simulink model "QRotorSimulation"  (R2023a)
settings: Solver=VariableStepAuto  StartTime=0.0  StopTime=100  RelTol=1e-9
values from neighbouring files (symbols this model uses):
  A = [-skew(Oc),   eye(3),        -skew(Vc), zeros(3), zeros(3,4) ... (first row only)    [diff_q.m]    (also in model_LQR_Obsever.m)
  B = [   [0;0;0],zeros(3) ... (first row only)    [diff_q.m]    (also in model_LQR_Obsever.m)
  C = [    eye(3),   zeros(3), zeros(3),  zeros(3),zeros(3,4) ... (first row only)    [diff_q.m]    (also in model_LQR_Obsever.m)
  k = lqr(A, B, Q, R)    [model_LQR_Obsever.m]
  k1 = lqr(A1, B1, Q1, R)    [diff_q.m]    (also in model_LQR_Obsever.m)
  L_acker = (place(A',C', desired_poles))'    [diff_q.m]    (also in model_LQR_Obsever.m)
  target_pos = [1,1,1]    [diff_q.m]
libraries: robotcorelib x1, uavutilslib x1
settings Model: PacingRate=79  Creator=carlossilvestre  LastModifiedBy=ADMIN
settings SolverCC: AlgebraicLoopSolver=TrustRegion
settings OptimizationCC: ReuseModelBlockBuffer=off
settings DebuggingCC: UnconnectedInputMsg=warning  UnconnectedOutputMsg=warning  UnconnectedLineMsg=warning
settings ModelReferenceCC: EnableRefExpFcnMdlSchedulingChecks=on

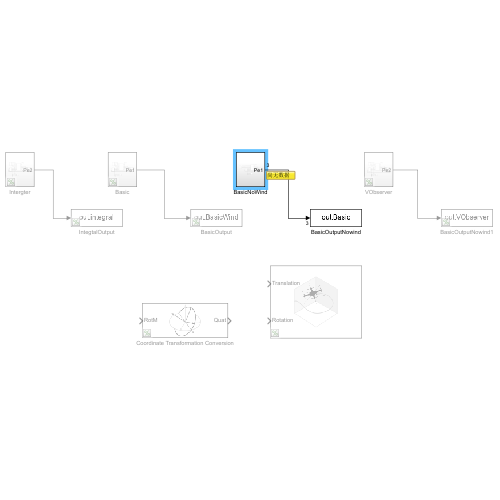
[thumbnail: Simulink's stored preview of the top-level diagram]
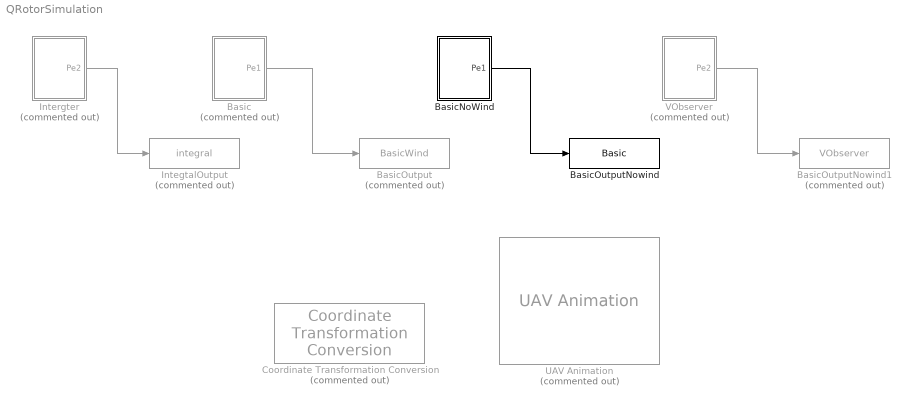
== system QRotorSimulation ==
  Basic : Subsystem  Commented=on
  BasicNoWind : Subsystem
  BasicOutput : ToWorkspace  Commented=on  VariableName=BasicWind  SaveFormat=Timeseries  SampleTime=-1
  BasicOutputNowind : ToWorkspace  VariableName=Basic  SaveFormat=Timeseries  SampleTime=-1
  BasicOutputNowind1 : ToWorkspace  Commented=on  VariableName=VObserver  SaveFormat=Timeseries  SampleTime=-1
  Coordinate Transformation Conversion : robotcorelib/Coordinate Transformation Conversion  Commented=on  InputRepresentation=Rotation Matrix  InputEulerSequence=ZYX  ShowTrVecInputPort=on  OutputRepresentation=Quaternion  OutputEulerSequence=ZYX  ShowTrVecOutputPort=on  SimulateUsing=Interpreted execution
      settings: LibrarySourceBlock=uavutilslib/Coordinate Transformation Conversion
  IntegtalOutput : ToWorkspace  Commented=on  VariableName=integral  SaveFormat=Timeseries  SampleTime=-1
  Intergter : Subsystem  Commented=on
  UAV Animation : uavutilslib/UAV Animation  Commented=on  UAVType=Multirotor  UAVSize=1  InertialZDirection=Down  SampleTime=-1
  VObserver : Subsystem  Commented=on
  wires:
  Intergter/1(Pe2) -> IntegtalOutput/1
  Basic/1(Pe1) -> BasicOutput/1
  BasicNoWind/1(Pe1) -> BasicOutputNowind/1
  VObserver/1(Pe2) -> BasicOutputNowind1/1

== system QRotorSimulation/Basic ==
  Constant : Constant  Value=k1
  Controller : Subsystem
  Demux : Demux  Outputs=3
  Nonlinear Transformation : MATLAB Function  TreatAsAtomicUnit=on
  Quardrotor : Subsystem
  Target Generator : Subsystem
  Ve : Scope
  XY Graph : Record  FileSettingsInternal="{\"entries\":[{\"content\":{\"excelSettings\":{\"content\":{},\"type\":\"Streamout.ExcelSettings\"}},\"type\":\"Streamout.FileSettingStorage\",\"uuid\":\"0487771f-67df-4d95-832c-7bf71d09cbca\"}],\"packageUris\":[\"http://schema.mathworks.com/mf0/streamout_blocks/R2020a\"],\"version\":\"1.0\"}"  Layout=[1 1]  SignalsInternal="{\"entries\":[{\"content\":{\"signals\":[{\"content\":{\"blockPath\":[\"QRotorSimulation/Basic/XY Graph\"],\"dimensions\":[1],\"domain\":\"QRotorSimulation/Basic/XY Graph\",\"lineColor\":\"#d95319\",\"port\":1,\"signalID\":1086,\"signalName\":\"Demux:1\"},\"type\":\"RecordBlkView.Signal\",\"uuid\":\"f90e91e6-e4ac-4811-9662-c694516e1994\"},{\"content\":{\"blockPath\":[\"QRotorSimulation/Basic/XY Graph\"],\"dimensions\":[1],\"domain\":\"QRotorSimulation/Basic/XY Graph\",\"lineColor\":\"#edb120\",\"port\":2,\"signalID\":1089,\"signalName\":\"Demux:2\"},\"type\":\"RecordBlkView.Signal\",\"uuid\":\"4a6e3aa6-85d4-4a9f-a4ee-96b742c40e35\"}]},\"type\":\"RecordBlkView.InputSignals\",\"uuid\":\"6a15db31-b281-48b1-89f1-5f9fae2ff927\"}],\"packageUris\":[\"http://schema.mathworks.com/mf0/streamout_blocks/R2020a\"],\"version\":\"1.0\"}"  VisualizationBindings="{\"xyplotplugin\":{\"info\":[{\"series\":[],\"subplotID\":1}]}}"  CompatibilityTag=XY
  Pe1 : Outport
  wires:
  Quardrotor/1(P) -> Demux/1, Pe1/1, Nonlinear Transformation/5(P)
  Quardrotor/3(Omega) -> Nonlinear Transformation/7(Omega)
  Nonlinear Transformation/3(Le) -> Controller/3(Le)
  Constant/1 -> Controller/5(k)
  Controller/2(T) -> Quardrotor/2(Thrust)
  Target Generator/4(Omega C) -> Nonlinear Transformation/3(OmeagC)
  Target Generator/5(R C) -> Nonlinear Transformation/4(Rc)
  Nonlinear Transformation/4(Pe) -> Controller/4(Pe)
  Nonlinear Transformation/1(Ve) -> Ve/1, Controller/1(Ve)
  Target Generator/2(Velocity C) -> Nonlinear Transformation/2(Vc)
  Quardrotor/2(V) -> Nonlinear Transformation/6(V)
  Nonlinear Transformation/2(Oe) -> Controller/2(Oe)
  Controller/1(n) -> Quardrotor/1(Torque)
  Target Generator/1(Position C) -> Nonlinear Transformation/1(Pc)
  Demux/2 -> XY Graph/2
  Demux/1 -> XY Graph/1
  Quardrotor/4(R) -> Nonlinear Transformation/8(R)

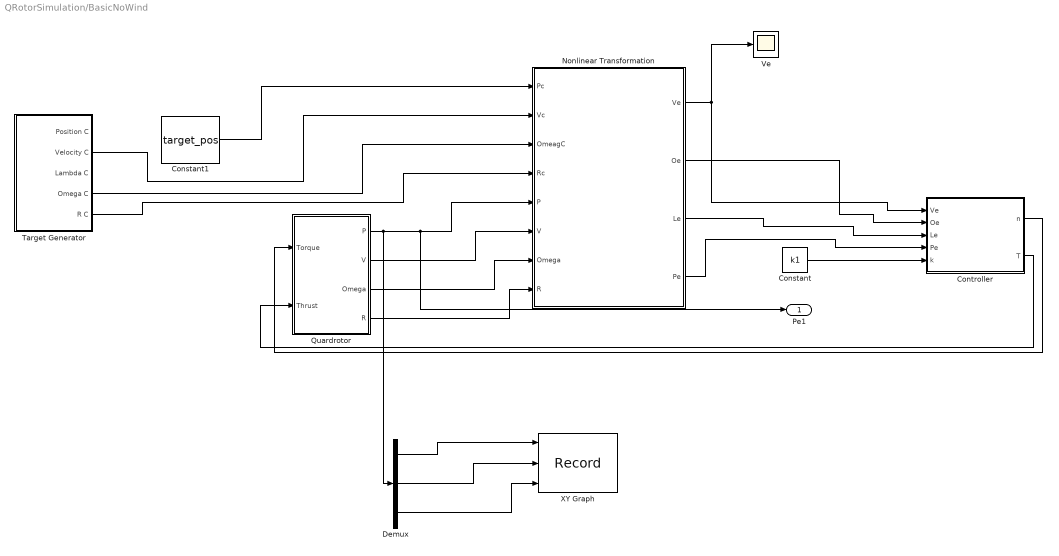
== system QRotorSimulation/BasicNoWind ==
  Constant : Constant  Value=k1
  Constant1 : Constant  Value=target_pos
  Controller : Subsystem
  Demux : Demux  Outputs=3
  Nonlinear Transformation : MATLAB Function  TreatAsAtomicUnit=on
  Quardrotor : Subsystem
  Target Generator : Subsystem
  Ve : Scope
  XY Graph : Record  FileSettingsInternal="{\"entries\":[{\"content\":{\"excelSettings\":{\"content\":{},\"type\":\"Streamout.ExcelSettings\"}},\"type\":\"Streamout.FileSettingStorage\",\"uuid\":\"6b954509-a0f9-4bc4-929f-937e6fe2c196\"}],\"packageUris\":[\"http://schema.mathworks.com/mf0/streamout_blocks/R2020a\"],\"version\":\"1.0\"}"  Layout=[1 1]  SignalsInternal="{\"entries\":[{\"content\":{\"signals\":[{\"content\":{\"blockPath\":[\"QRotorSimulation/BasicNoWind/XY Graph\"],\"dimensions\":[1],\"domain\":\"QRotorSimulation/BasicNoWind/XY Graph\",\"lineColor\":\"#77ac30\",\"port\":1,\"sid\":[\"\"],\"signalID\":3826,\"signalName\":\"Demux:1\"},\"type\":\"RecordBlkView.Signal\",\"uuid\":\"1b7d485a-109d-4aad-9f55-56817bc70bf2\"},{\"content\":{\"blockPath\":[\"QRotorSimulation/BasicNoWind/XY Graph\"],\"dimensions\":[1],\"domain\":\"QRotorSimulation/BasicNoWind/XY Graph\",\"lineColor\":\"#4dbeee\",\"port\":2,\"sid\":[\"\"],\"signalID\":3830,\"signalName\":\"Demux:2\"},\"type\":\"RecordBlkView.Signal\",\"uuid\":\"83925266-2204-43e3-9e67-c8fa90e0486b\"},{\"content\":{\"blockPath\":[\"QRotorSimulation/BasicNoWind/XY Graph\"],\"dimensions\":[1],\"domain\":\"QRotorSimulation/BasicNoWind/XY Graph\",\"lineColor\":\"#a2142f\",\"port\":3,\"sid\":[\"\"],\"signalID\":3834,\"signalName\":\"Demux:3\"},\"type\":\"RecordBlkView.Signal\",\"uuid\":\"81f905cc-e198-402a-a94e-d97bcbf9668d\"}]},\"type\":\"RecordBlkView.InputSignals\",\"uuid\":\"1cf66a60-863d-452f-b7c5-5f047e404abc\"}],\"packageUris\":[\"http://schema.mathworks.com/mf0/streamout_blocks/R2020a\"],\"version\":\"1.0\"}"  VisualizationBindings="{\"xyplotplugin\":{\"info\":[{\"series\":[],\"subplotID\":1}]}}"  CompatibilityTag=XY
  Pe1 : Outport
  wires:
  Quardrotor/4(R) -> Nonlinear Transformation/8(R)
  Demux/1 -> XY Graph/1
  Demux/2 -> XY Graph/2
  Controller/1(n) -> Quardrotor/1(Torque)
  Nonlinear Transformation/2(Oe) -> Controller/2(Oe)
  Quardrotor/2(V) -> Nonlinear Transformation/6(V)
  Target Generator/2(Velocity C) -> Nonlinear Transformation/2(Vc)
  Nonlinear Transformation/1(Ve) -> Controller/1(Ve), Ve/1
  Nonlinear Transformation/4(Pe) -> Controller/4(Pe)
  Target Generator/5(R C) -> Nonlinear Transformation/4(Rc)
  Target Generator/4(Omega C) -> Nonlinear Transformation/3(OmeagC)
  Controller/2(T) -> Quardrotor/2(Thrust)
  Constant/1 -> Controller/5(k)
  Nonlinear Transformation/3(Le) -> Controller/3(Le)
  Quardrotor/3(Omega) -> Nonlinear Transformation/7(Omega)
  Quardrotor/1(P) -> Pe1/1, Nonlinear Transformation/5(P), Demux/1
  Demux/3 -> XY Graph/3
  Constant1/1 -> Nonlinear Transformation/1(Pc)

== system QRotorSimulation/Intergter ==
  Constant : Constant  Value=k
  Controller : Subsystem
  Demux : Demux  Outputs=3
  Nonlinear Transformation : MATLAB Function  TreatAsAtomicUnit=on
  Pe : Scope
  Quardrotor : Subsystem
  Target Generator : Subsystem
  Ve : Scope
  XY Graph : Record  FileSettingsInternal="{\"entries\":[{\"content\":{\"excelSettings\":{\"content\":{},\"type\":\"Streamout.ExcelSettings\"}},\"type\":\"Streamout.FileSettingStorage\",\"uuid\":\"5274d8c0-192d-4b89-88ac-329a06cc1ef7\"}],\"packageUris\":[\"http://schema.mathworks.com/mf0/streamout_blocks/R2020a\"],\"version\":\"1.0\"}"  Layout=[1 1]  SignalsInternal="{\"entries\":[{\"content\":{\"signals\":[{\"content\":{\"blockPath\":[\"QRotorSimulation/Intergter/XY Graph\"],\"dimensions\":[1],\"domain\":\"QRotorSimulation/Intergter/XY Graph\",\"lineColor\":\"#64d413\",\"port\":1,\"signalID\":1070,\"signalName\":\"Demux:1\"},\"type\":\"RecordBlkView.Signal\",\"uuid\":\"1ff87784-21ca-461c-803a-48280af1891b\"},{\"content\":{\"blockPath\":[\"QRotorSimulation/Intergter/XY Graph\"],\"dimensions\":[1],\"domain\":\"QRotorSimulation/Intergter/XY Graph\",\"lineColor\":\"#ff13a6\",\"port\":2,\"signalID\":1073,\"signalName\":\"Demux:2\"},\"type\":\"RecordBlkView.Signal\",\"uuid\":\"24908c8c-4281-4163-98ae-854703be901d\"}]},\"type\":\"RecordBlkView.InputSignals\",\"uuid\":\"2df63969-910d-47c6-a209-6b5a32245b9d\"}],\"packageUris\":[\"http://schema.mathworks.com/mf0/streamout_blocks/R2020a\"],\"version\":\"1.0\"}"  VisualizationBindings="{\"xyplotplugin\":{\"info\":[{\"series\":[],\"subplotID\":1}]}}"  CompatibilityTag=XY
  Pe2 : Outport
  wires:
  Quardrotor/4(R) -> Nonlinear Transformation/8(R)
  Demux/1 -> XY Graph/1
  Demux/2 -> XY Graph/2
  Target Generator/1(Position C) -> Nonlinear Transformation/1(Pc)
  Controller/1(n) -> Quardrotor/1(Torque)
  Nonlinear Transformation/2(Oe) -> Controller/2(Oe)
  Quardrotor/2(V) -> Nonlinear Transformation/6(V)
  Target Generator/2(Velocity C) -> Nonlinear Transformation/2(Vc)
  Nonlinear Transformation/1(Ve) -> Controller/1(Ve), Ve/1
  Target Generator/5(R C) -> Nonlinear Transformation/4(Rc)
  Target Generator/4(Omega C) -> Nonlinear Transformation/3(OmeagC)
  Controller/2(T) -> Quardrotor/2(Thrust)
  Constant/1 -> Controller/5(k)
  Nonlinear Transformation/3(Le) -> Controller/3(Le)
  Quardrotor/3(Omega) -> Nonlinear Transformation/7(Omega)
  Quardrotor/1(P) -> Nonlinear Transformation/5(P), Pe2/1, Demux/1
  Nonlinear Transformation/4(Pe) -> Controller/4(Pe), Pe/1

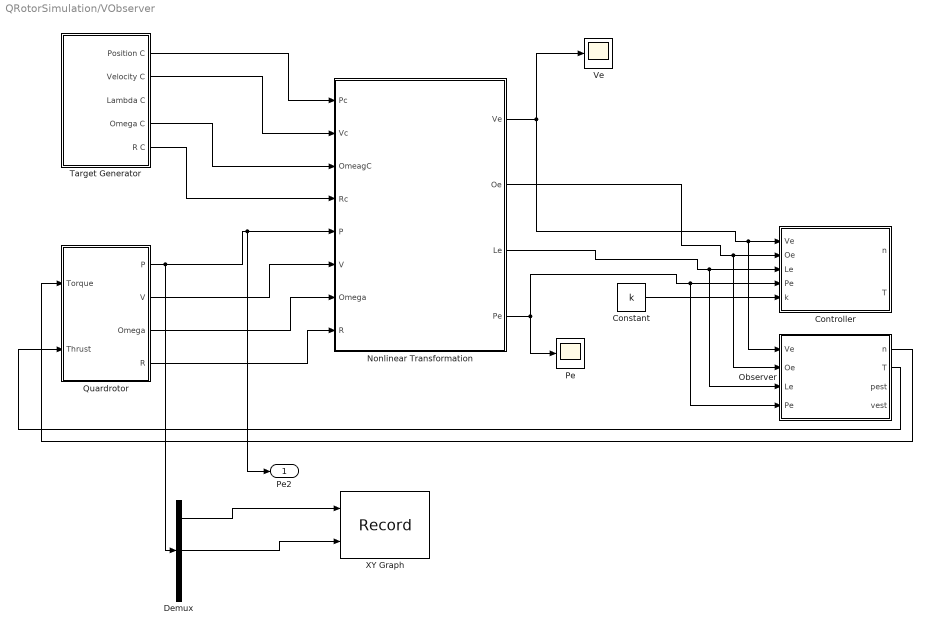
== system QRotorSimulation/VObserver ==
  Constant : Constant  Value=k
  Controller : Subsystem
  Demux : Demux  Outputs=3
  Nonlinear Transformation : MATLAB Function  TreatAsAtomicUnit=on
  Observer : Subsystem
  Pe : Scope
  Quardrotor : Subsystem
  Target Generator : Subsystem
  Ve : Scope
  XY Graph : Record  FileSettingsInternal="{\"entries\":[{\"content\":{\"excelSettings\":{\"content\":{},\"type\":\"Streamout.ExcelSettings\"}},\"type\":\"Streamout.FileSettingStorage\",\"uuid\":\"09f89506-ea5c-4e7c-be6e-909bc9330a96\"}],\"packageUris\":[\"http://schema.mathworks.com/mf0/streamout_blocks/R2020a\"],\"version\":\"1.0\"}"  Layout=[1 1]  SignalsInternal="{\"entries\":[{\"content\":{\"signals\":[{\"content\":{\"blockPath\":[\"QRotorSimulation/VObserver/XY Graph\"],\"dimensions\":[1],\"domain\":\"QRotorSimulation/VObserver/XY Graph\",\"lineColor\":\"#7e2f8e\",\"port\":1,\"signalID\":1062,\"signalName\":\"Demux:1\"},\"type\":\"RecordBlkView.Signal\",\"uuid\":\"913ab4c1-d204-4348-ad14-4cd9366a4f4d\"},{\"content\":{\"blockPath\":[\"QRotorSimulation/VObserver/XY Graph\"],\"dimensions\":[1],\"domain\":\"QRotorSimulation/VObserver/XY Graph\",\"lineColor\":\"#77ac30\",\"port\":2,\"signalID\":1065,\"signalName\":\"Demux:2\"},\"type\":\"RecordBlkView.Signal\",\"uuid\":\"1419c895-5134-46cb-881d-871a74845bf3\"}]},\"type\":\"RecordBlkView.InputSignals\",\"uuid\":\"c0c07795-0499-4d5b-ba90-fdcac508c0e4\"}],\"packageUris\":[\"http://schema.mathworks.com/mf0/streamout_blocks/R2020a\"],\"version\":\"1.0\"}"  VisualizationBindings="{\"xyplotplugin\":{\"info\":[{\"series\":[],\"subplotID\":1}]}}"  CompatibilityTag=XY
  Pe2 : Outport
  wires:
  Nonlinear Transformation/4(Pe) -> Pe/1, Observer/4(Pe), Controller/4(Pe)
  Quardrotor/1(P) -> Demux/1, Pe2/1, Nonlinear Transformation/5(P)
  Quardrotor/3(Omega) -> Nonlinear Transformation/7(Omega)
  Nonlinear Transformation/3(Le) -> Observer/3(Le), Controller/3(Le)
  Constant/1 -> Controller/5(k)
  Target Generator/4(Omega C) -> Nonlinear Transformation/3(OmeagC)
  Target Generator/5(R C) -> Nonlinear Transformation/4(Rc)
  Nonlinear Transformation/1(Ve) -> Ve/1, Observer/1(Ve), Controller/1(Ve)
  Target Generator/2(Velocity C) -> Nonlinear Transformation/2(Vc)
  Quardrotor/2(V) -> Nonlinear Transformation/6(V)
  Nonlinear Transformation/2(Oe) -> Observer/2(Oe), Controller/2(Oe)
  Target Generator/1(Position C) -> Nonlinear Transformation/1(Pc)
  Demux/2 -> XY Graph/2
  Demux/1 -> XY Graph/1
  Quardrotor/4(R) -> Nonlinear Transformation/8(R)
  Observer/1(n) -> Quardrotor/1(Torque)
  Observer/2(T) -> Quardrotor/2(Thrust)

== system QRotorSimulation/Basic/Controller ==
  Ve : Inport
  Oe : Inport  Port=2
  Le : Inport  Port=3
  Pe : Inport  Port=4
  k : Inport  Port=5
  Controller : MATLAB Function  TreatAsAtomicUnit=on
  n : Outport
  T : Outport  Port=2
  wires:
  Oe/1 -> Controller/2(Oe)
  Pe/1 -> Controller/4(Pe)
  Le/1 -> Controller/3(Le)
  Ve/1 -> Controller/1(Ve)
  Controller/2(n) -> n/1
  k/1 -> Controller/5(k)
  Controller/1(T) -> T/1

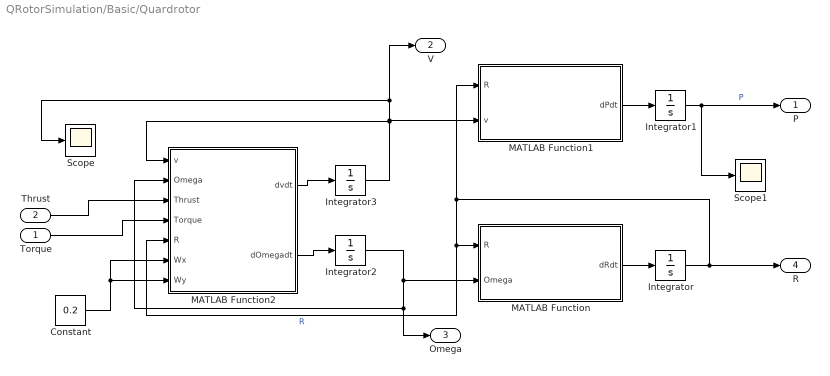
== system QRotorSimulation/Basic/Quardrotor ==
  Torque : Inport
  Thrust : Inport  Port=2  PortDimensions=1
  Constant : Constant  Value=0.2  VectorParams1D=off
  Integrator : Integrator  InitialCondition=eye(3)
  Integrator1 : Integrator  InitialCondition=[0,0,0]
  Integrator2 : Integrator  InitialCondition=[0,0,0]  ContinuousStateAttributes='omega'
  Integrator3 : Integrator  InitialCondition=[0,0,0]  ContinuousStateAttributes='velocity'
  MATLAB Function : MATLAB Function  TreatAsAtomicUnit=on
  MATLAB Function1 : MATLAB Function  TreatAsAtomicUnit=on
  MATLAB Function2 : MATLAB Function  TreatAsAtomicUnit=on
  Scope : Scope
  Scope1 : Scope
  P : Outport
  V : Outport  Port=2
  Omega : Outport  Port=3
  R : Outport  Port=4
  wires:
  Constant/1 -> MATLAB Function2/6(Wx), MATLAB Function2/7(Wy)
  Torque/1 -> MATLAB Function2/4(Torque)
  Thrust/1 -> MATLAB Function2/3(Thrust)
  Integrator/1 -> MATLAB Function/1(R), MATLAB Function2/5(R), MATLAB Function1/1(R), R/1  "R"
  MATLAB Function1/1(dPdt) -> Integrator1/1
  Integrator3/1 -> MATLAB Function2/1(v), MATLAB Function1/2(v), V/1, Scope/1
  MATLAB Function2/2(dOmegadt) -> Integrator2/1
  MATLAB Function/1(dRdt) -> Integrator/1
  Integrator2/1 -> MATLAB Function/2(Omega), MATLAB Function2/2(Omega), Omega/1
  Integrator1/1 -> P/1, Scope1/1  "P"
  MATLAB Function2/1(dvdt) -> Integrator3/1

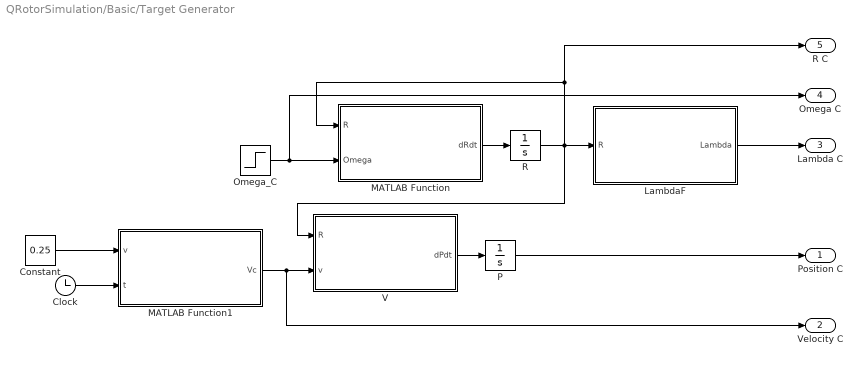
== system QRotorSimulation/Basic/Target Generator ==
  Clock : Clock
  Constant : Constant  Value=0.25
  LambdaF : MATLAB Function  TreatAsAtomicUnit=on
  MATLAB Function : MATLAB Function  TreatAsAtomicUnit=on
  MATLAB Function1 : MATLAB Function  TreatAsAtomicUnit=on
  Omega_C : Step  Time=0  Before=[0;0;0]  After=[0;0;0]  SampleTime=0
  P : Integrator
  R : Integrator  InitialCondition=eye(3)
  V : MATLAB Function  TreatAsAtomicUnit=on
  Position C : Outport
  Velocity C : Outport  Port=2
  Lambda C : Outport  Port=3
  Omega C : Outport  Port=4
  R C : Outport  Port=5
  wires:
  Clock/1 -> MATLAB Function1/2(t)
  Constant/1 -> MATLAB Function1/1(v)
  Omega_C/1 -> MATLAB Function/2(Omega), Omega C/1
  MATLAB Function1/1(Vc) -> V/2(v), Velocity C/1
  V/1(dPdt) -> P/1
  R/1 -> LambdaF/1(R), V/1(R), R C/1, MATLAB Function/1(R)
  MATLAB Function/1(dRdt) -> R/1
  P/1 -> Position C/1
  LambdaF/1(Lambda) -> Lambda C/1

== system QRotorSimulation/BasicNoWind/Controller ==
  Ve : Inport
  Oe : Inport  Port=2
  Le : Inport  Port=3
  Pe : Inport  Port=4
  k : Inport  Port=5
  Controller : MATLAB Function  TreatAsAtomicUnit=on
  n : Outport
  T : Outport  Port=2
  wires:
  Controller/1(T) -> T/1
  k/1 -> Controller/5(k)
  Controller/2(n) -> n/1
  Ve/1 -> Controller/1(Ve)
  Le/1 -> Controller/3(Le)
  Pe/1 -> Controller/4(Pe)
  Oe/1 -> Controller/2(Oe)

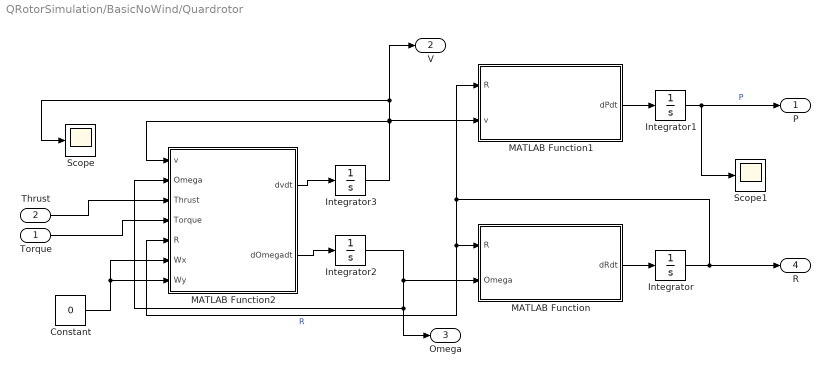
== system QRotorSimulation/BasicNoWind/Quardrotor ==
  Torque : Inport
  Thrust : Inport  Port=2  PortDimensions=1
  Constant : Constant  Value=0  VectorParams1D=off
  Integrator : Integrator  InitialCondition=eye(3)
  Integrator1 : Integrator  InitialCondition=[0,0,0]
  Integrator2 : Integrator  InitialCondition=[0,0,0]  ContinuousStateAttributes='omega'
  Integrator3 : Integrator  InitialCondition=[0,0,0]  ContinuousStateAttributes='velocity'
  MATLAB Function : MATLAB Function  TreatAsAtomicUnit=on
  MATLAB Function1 : MATLAB Function  TreatAsAtomicUnit=on
  MATLAB Function2 : MATLAB Function  TreatAsAtomicUnit=on
  Scope : Scope
  Scope1 : Scope
  P : Outport
  V : Outport  Port=2
  Omega : Outport  Port=3
  R : Outport  Port=4
  wires:
  MATLAB Function2/1(dvdt) -> Integrator3/1
  Integrator1/1 -> Scope1/1, P/1  "P"
  Integrator2/1 -> Omega/1, MATLAB Function2/2(Omega), MATLAB Function/2(Omega)
  MATLAB Function/1(dRdt) -> Integrator/1
  MATLAB Function2/2(dOmegadt) -> Integrator2/1
  Integrator3/1 -> Scope/1, V/1, MATLAB Function1/2(v), MATLAB Function2/1(v)
  MATLAB Function1/1(dPdt) -> Integrator1/1
  Integrator/1 -> R/1, MATLAB Function1/1(R), MATLAB Function2/5(R), MATLAB Function/1(R)  "R"
  Thrust/1 -> MATLAB Function2/3(Thrust)
  Torque/1 -> MATLAB Function2/4(Torque)
  Constant/1 -> MATLAB Function2/7(Wy), MATLAB Function2/6(Wx)

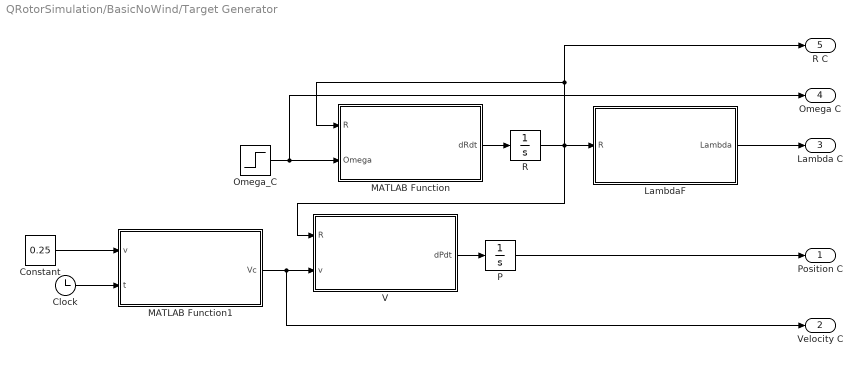
== system QRotorSimulation/BasicNoWind/Target Generator ==
  Clock : Clock
  Constant : Constant  Value=0.25
  LambdaF : MATLAB Function  TreatAsAtomicUnit=on
  MATLAB Function : MATLAB Function  TreatAsAtomicUnit=on
  MATLAB Function1 : MATLAB Function  TreatAsAtomicUnit=on
  Omega_C : Step  Time=0  Before=[0;0;0]  After=[0;0;0]  SampleTime=0
  P : Integrator
  R : Integrator  InitialCondition=eye(3)
  V : MATLAB Function  TreatAsAtomicUnit=on
  Position C : Outport
  Velocity C : Outport  Port=2
  Lambda C : Outport  Port=3
  Omega C : Outport  Port=4
  R C : Outport  Port=5
  wires:
  LambdaF/1(Lambda) -> Lambda C/1
  P/1 -> Position C/1
  MATLAB Function/1(dRdt) -> R/1
  R/1 -> MATLAB Function/1(R), R C/1, V/1(R), LambdaF/1(R)
  V/1(dPdt) -> P/1
  MATLAB Function1/1(Vc) -> Velocity C/1, V/2(v)
  Omega_C/1 -> Omega C/1, MATLAB Function/2(Omega)
  Constant/1 -> MATLAB Function1/1(v)
  Clock/1 -> MATLAB Function1/2(t)

== system QRotorSimulation/Intergter/Controller ==
  Ve : Inport
  Oe : Inport  Port=2
  Le : Inport  Port=3
  Pe : Inport  Port=4
  k : Inport  Port=5
  Controller : MATLAB Function  TreatAsAtomicUnit=on
  Int : MATLAB Function  TreatAsAtomicUnit=on
  Integrator : Integrator
  n : Outport
  T : Outport  Port=2
  wires:
  Controller/1(T) -> T/1
  k/1 -> Controller/6(k)
  Controller/2(n) -> n/1
  Integrator/1 -> Controller/5(Xi)
  Int/1(dXidt) -> Integrator/1
  Ve/1 -> Int/1(Ve), Controller/1(Ve)
  Le/1 -> Controller/3(Le), Int/3(Le)
  Pe/1 -> Controller/4(Pe), Int/4(Pe)
  Oe/1 -> Int/2(Oe), Controller/2(Oe)

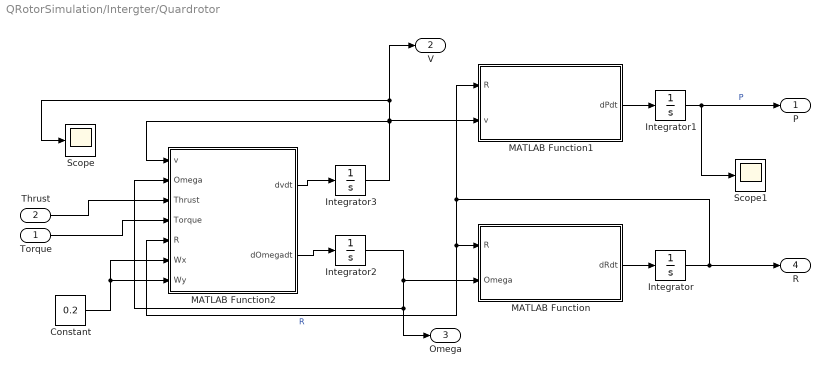
== system QRotorSimulation/Intergter/Quardrotor ==
  Torque : Inport
  Thrust : Inport  Port=2  PortDimensions=1
  Constant : Constant  Value=0.2
  Integrator : Integrator  InitialCondition=eye(3)
  Integrator1 : Integrator  InitialCondition=[0,0,0]
  Integrator2 : Integrator  InitialCondition=[0,0,0]  ContinuousStateAttributes='omega'
  Integrator3 : Integrator  InitialCondition=[0,0,0]  ContinuousStateAttributes='velocity'
  MATLAB Function : MATLAB Function  TreatAsAtomicUnit=on
  MATLAB Function1 : MATLAB Function  TreatAsAtomicUnit=on
  MATLAB Function2 : MATLAB Function  TreatAsAtomicUnit=on
  Scope : Scope
  Scope1 : Scope
  P : Outport
  V : Outport  Port=2
  Omega : Outport  Port=3
  R : Outport  Port=4
  wires:
  MATLAB Function2/1(dvdt) -> Integrator3/1
  Integrator1/1 -> Scope1/1, P/1  "P"
  Integrator2/1 -> Omega/1, MATLAB Function2/2(Omega), MATLAB Function/2(Omega)
  MATLAB Function/1(dRdt) -> Integrator/1
  MATLAB Function2/2(dOmegadt) -> Integrator2/1
  Integrator3/1 -> Scope/1, V/1, MATLAB Function1/2(v), MATLAB Function2/1(v)
  MATLAB Function1/1(dPdt) -> Integrator1/1
  Integrator/1 -> R/1, MATLAB Function1/1(R), MATLAB Function2/5(R), MATLAB Function/1(R)  "R"
  Thrust/1 -> MATLAB Function2/3(Thrust)
  Torque/1 -> MATLAB Function2/4(Torque)
  Constant/1 -> MATLAB Function2/7(Wy), MATLAB Function2/6(Wx)

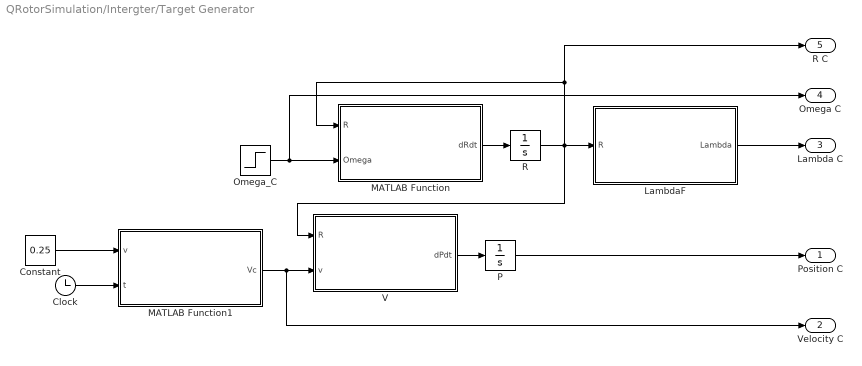
== system QRotorSimulation/Intergter/Target Generator ==
  Clock : Clock
  Constant : Constant  Value=0.25
  LambdaF : MATLAB Function  TreatAsAtomicUnit=on
  MATLAB Function : MATLAB Function  TreatAsAtomicUnit=on
  MATLAB Function1 : MATLAB Function  TreatAsAtomicUnit=on
  Omega_C : Step  Time=0  Before=[0;0;0]  After=[0;0;0]  SampleTime=0
  P : Integrator
  R : Integrator  InitialCondition=eye(3)
  V : MATLAB Function  TreatAsAtomicUnit=on
  Position C : Outport
  Velocity C : Outport  Port=2
  Lambda C : Outport  Port=3
  Omega C : Outport  Port=4
  R C : Outport  Port=5
  wires:
  LambdaF/1(Lambda) -> Lambda C/1
  P/1 -> Position C/1
  MATLAB Function/1(dRdt) -> R/1
  R/1 -> MATLAB Function/1(R), R C/1, V/1(R), LambdaF/1(R)
  V/1(dPdt) -> P/1
  MATLAB Function1/1(Vc) -> Velocity C/1, V/2(v)
  Omega_C/1 -> Omega C/1, MATLAB Function/2(Omega)
  Constant/1 -> MATLAB Function1/1(v)
  Clock/1 -> MATLAB Function1/2(t)

== system QRotorSimulation/VObserver/Controller ==
  Ve : Inport
  Oe : Inport  Port=2
  Le : Inport  Port=3
  Pe : Inport  Port=4
  k : Inport  Port=5
  Controller : MATLAB Function  TreatAsAtomicUnit=on
  Int : MATLAB Function  TreatAsAtomicUnit=on
  Integrator : Integrator
  n : Outport
  T : Outport  Port=2
  wires:
  Oe/1 -> Controller/2(Oe), Int/2(Oe)
  Pe/1 -> Int/4(Pe), Controller/4(Pe)
  Le/1 -> Int/3(Le), Controller/3(Le)
  Ve/1 -> Controller/1(Ve), Int/1(Ve)
  Int/1(dXidt) -> Integrator/1
  Integrator/1 -> Controller/5(Xi)
  Controller/2(n) -> n/1
  k/1 -> Controller/6(k)
  Controller/1(T) -> T/1

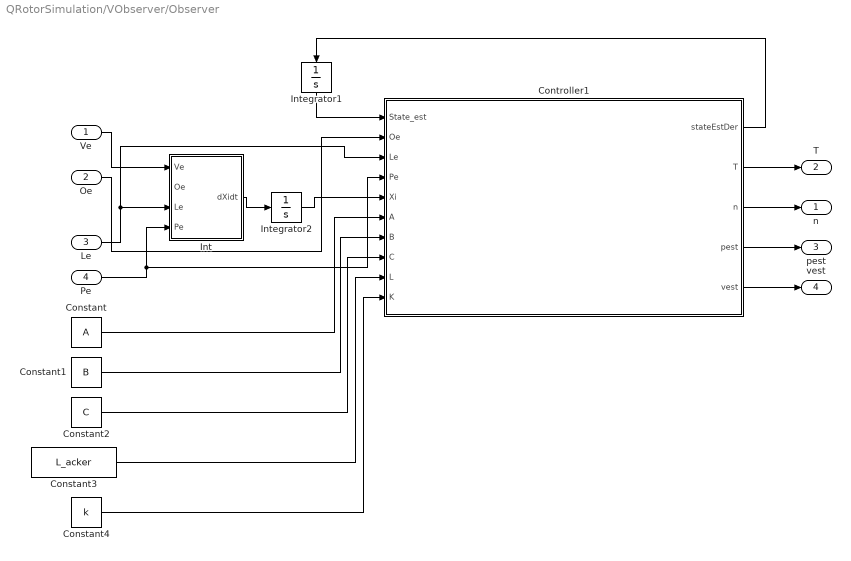
== system QRotorSimulation/VObserver/Observer ==
  Ve : Inport
  Oe : Inport  Port=2
  Le : Inport  Port=3
  Pe : Inport  Port=4
  Constant : Constant  Value=A
  Constant1 : Constant  Value=B
  Constant2 : Constant  Value=C
  Constant3 : Constant  Value=L_acker
  Constant4 : Constant  Value=k
  Controller1 : MATLAB Function  TreatAsAtomicUnit=on
  Int : MATLAB Function  TreatAsAtomicUnit=on
  Integrator1 : Integrator  InitialCondition=zeros(16,1)
  Integrator2 : Integrator
  n : Outport
  T : Outport  Port=2
  pest : Outport  Port=3
  vest : Outport  Port=4
  wires:
  Integrator1/1 -> Controller1/1(State_est)
  Controller1/1(stateEstDer) -> Integrator1/1
  Oe/1 -> Controller1/2(Oe)
  Pe/1 -> Controller1/4(Pe), Int/4(Pe)
  Le/1 -> Controller1/3(Le), Int/3(Le)
  Int/1(dXidt) -> Integrator2/1
  Controller1/2(T) -> T/1
  Controller1/3(n) -> n/1
  Constant/1 -> Controller1/6(A)
  Constant1/1 -> Controller1/7(B)
  Constant2/1 -> Controller1/8(C)
  Constant4/1 -> Controller1/10(K)
  Constant3/1 -> Controller1/9(L)
  Integrator2/1 -> Controller1/5(Xi)
  Controller1/5(vest) -> vest/1
  Controller1/4(pest) -> pest/1
  Ve/1 -> Int/1(Ve)

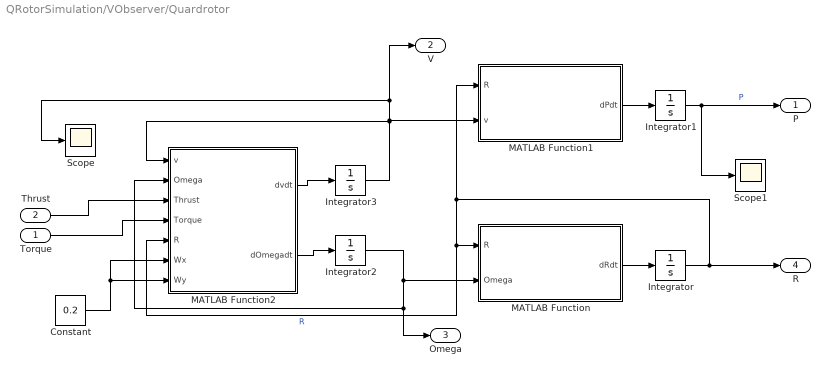
== system QRotorSimulation/VObserver/Quardrotor ==
  Torque : Inport
  Thrust : Inport  Port=2  PortDimensions=1
  Constant : Constant  Value=0.2
  Integrator : Integrator  InitialCondition=eye(3)
  Integrator1 : Integrator  InitialCondition=[0,0,0]
  Integrator2 : Integrator  InitialCondition=[0,0,0]  ContinuousStateAttributes='omega'
  Integrator3 : Integrator  InitialCondition=[0,0,0]  ContinuousStateAttributes='velocity'
  MATLAB Function : MATLAB Function  TreatAsAtomicUnit=on
  MATLAB Function1 : MATLAB Function  TreatAsAtomicUnit=on
  MATLAB Function2 : MATLAB Function  TreatAsAtomicUnit=on
  Scope : Scope
  Scope1 : Scope
  P : Outport
  V : Outport  Port=2
  Omega : Outport  Port=3
  R : Outport  Port=4
  wires:
  Constant/1 -> MATLAB Function2/6(Wx), MATLAB Function2/7(Wy)
  Torque/1 -> MATLAB Function2/4(Torque)
  Thrust/1 -> MATLAB Function2/3(Thrust)
  Integrator/1 -> MATLAB Function/1(R), MATLAB Function2/5(R), MATLAB Function1/1(R), R/1  "R"
  MATLAB Function1/1(dPdt) -> Integrator1/1
  Integrator3/1 -> MATLAB Function2/1(v), MATLAB Function1/2(v), V/1, Scope/1
  MATLAB Function2/2(dOmegadt) -> Integrator2/1
  MATLAB Function/1(dRdt) -> Integrator/1
  Integrator2/1 -> MATLAB Function/2(Omega), MATLAB Function2/2(Omega), Omega/1
  Integrator1/1 -> P/1, Scope1/1  "P"
  MATLAB Function2/1(dvdt) -> Integrator3/1

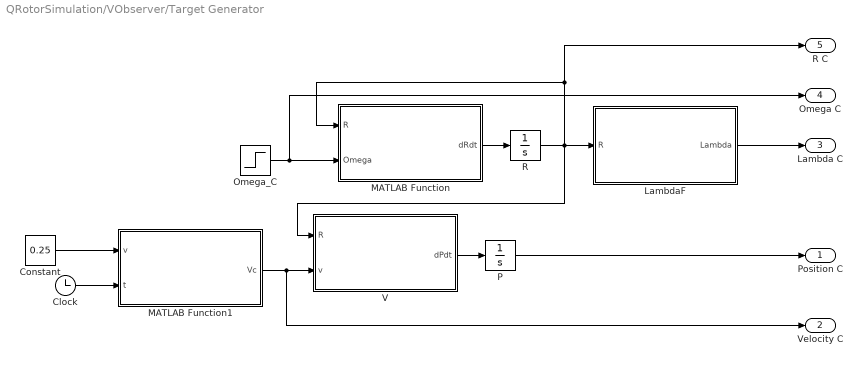
== system QRotorSimulation/VObserver/Target Generator ==
  Clock : Clock
  Constant : Constant  Value=0.25
  LambdaF : MATLAB Function  TreatAsAtomicUnit=on
  MATLAB Function : MATLAB Function  TreatAsAtomicUnit=on
  MATLAB Function1 : MATLAB Function  TreatAsAtomicUnit=on
  Omega_C : Step  Time=0  Before=[0;0;0]  After=[0;0;0]  SampleTime=0
  P : Integrator
  R : Integrator  InitialCondition=eye(3)
  V : MATLAB Function  TreatAsAtomicUnit=on
  Position C : Outport
  Velocity C : Outport  Port=2
  Lambda C : Outport  Port=3
  Omega C : Outport  Port=4
  R C : Outport  Port=5
  wires:
  Clock/1 -> MATLAB Function1/2(t)
  Constant/1 -> MATLAB Function1/1(v)
  Omega_C/1 -> MATLAB Function/2(Omega), Omega C/1
  MATLAB Function1/1(Vc) -> V/2(v), Velocity C/1
  V/1(dPdt) -> P/1
  R/1 -> LambdaF/1(R), V/1(R), R C/1, MATLAB Function/1(R)
  MATLAB Function/1(dRdt) -> R/1
  P/1 -> Position C/1
  LambdaF/1(Lambda) -> Lambda C/1

== matlab function QRotorSimulation/Intergter/Target Generator/MATLAB Function ==
  data: R input; dRdt output; Omega input
function dRdt = CompdRdt(R,Omega)
dRdt=R*skew(Omega);
end

== matlab function QRotorSimulation/Intergter/Target Generator/MATLAB Function1 ==
  data: v input; Vc output; t input
function Vc = VcGen(v,t)
Vc = [0;0;0];

if(t>10)
    Vc = [v;0;0];
end
if(t>30)
    Vc = [0;v;0];
end

if(t>50)
    Vc = [-v;0;0];
end

if(t>70)
    Vc = [0;-v;0]; 
end

if(t>90)
    Vc = [0;0;0]; %stop
end

end

== matlab function QRotorSimulation/Basic/Controller/Controller ==
  data: Ve input; Oe input; Le input; Pe input; T output; n output; k input
function [T,n] = Controller(Ve,Oe,Le,Pe,k)

State = [Pe; Ve; Le; Oe];
Cntl = -k * State;
T = Cntl(1);
n = Cntl(2:4);


end

== matlab function QRotorSimulation/BasicNoWind/Controller/Controller ==
  data: Ve input; Oe input; Le input; Pe input; T output; n output; k input
function [T,n] = Controller(Ve,Oe,Le,Pe,k)

State = [Pe; Ve; Le; Oe];
Cntl = -k * State;
T = Cntl(1);
n = Cntl(2:4);


end

== matlab function QRotorSimulation/Intergter/Controller/Int ==
  data: Ve input; Oe input; Le input; Pe input; dXidt output
function dXidt  = Intstate(Ve,Oe,Le,Pe)
dXidt = [Pe;Le(3)];



end

== matlab function QRotorSimulation/Basic/Nonlinear Transformation ==
  data: Pc input; Vc input; OmeagC input; Rc input; P input; V input; Omega input; R input; Ve output; Oe output; Le output; Pe output
function [Ve,Oe,Le,Pe] = Nonlinear_Transformation(Pc,Vc,OmeagC,Rc,P,V,Omega,R)

Ve = V - Vc;
Oe = Omega - OmeagC;
Pe = P - Pc;
Re = R * Rc';

Pitch = atan2(-Re(3,1),sqrt(Re(1,1)^2 + Re(2,1)^2));
Yaw = atan2(Re(2,1)/cos(Pitch),Re(1,1)/cos(Pitch));
Roll = atan2(Re(3,2)/cos(Pitch),Re(3,3)/cos(Pitch));
Le = [Roll;Pitch;Yaw];

end

== matlab function QRotorSimulation/Basic/Quardrotor/MATLAB Function ==
  data: R input; dRdt output; Omega input
function dRdt = CompdRdt(R,Omega)
dRdt=R*skew(Omega);
end

== matlab function QRotorSimulation/Basic/Quardrotor/MATLAB Function1 ==
  data: R input; dPdt output; v input
function dPdt = CompdPdt(R,v)
dPdt=R*v;
end

== matlab function QRotorSimulation/Basic/Quardrotor/MATLAB Function2 ==
  data: v input; Omega input; dvdt output; Thrust input; Torque input; dOmegadt output; R input; Wx input; Wy input
function [dvdt,dOmegadt] = Dynamics(v,Omega,Thrust,Torque,R,Wx,Wy)

m = 0.25;
g = 9.8;
I = 0.1 * eye(3);
Wind = [Wx;Wy;0];
F = - Thrust * [0;0;1] + m * g * R'*[0;0;1] + Wind;


dvdt = -skew(Omega)*v + 1/m * F;
dOmegadt = -I^-1 * skew(Omega) * I * Omega + I^-1 * Torque ;

end

== matlab function QRotorSimulation/Basic/Target Generator/LambdaF ==
  data: R input; Lambda output
function Lambda = R_to_Lambda(R)

Pitch = atan2(-R(3,1),sqrt(R(1,1)^2 + R(2,1)^2));
Yaw = atan2(R(2,1)/cos(Pitch),R(1,1)/cos(Pitch));
Roll = atan2(R(3,2)/cos(Pitch),R(3,3)/cos(Pitch));
Lambda = [Roll;Pitch;Yaw];

end

== matlab function QRotorSimulation/Basic/Target Generator/MATLAB Function ==
  data: R input; dRdt output; Omega input
function dRdt = CompdRdt(R,Omega)
dRdt=R*skew(Omega);
end

== matlab function QRotorSimulation/Basic/Target Generator/MATLAB Function1 ==
  data: v input; Vc output; t input
function Vc = VcGen(v,t)
Vc = [0;0;0];

if(t>10)
    Vc = [v;0;0];
end
if(t>30)
    Vc = [0;v;0];
end

if(t>50)
    Vc = [-v;0;0];
end

if(t>70)
    Vc = [0;-v;0]; 
end

if(t>90)
    Vc = [0;0;0]; %stop
end

end

== matlab function QRotorSimulation/Basic/Target Generator/V ==
  data: R input; dPdt output; v input
function dPdt = CompdPdt(R,v)
dPdt=R*v;
end

== matlab function QRotorSimulation/BasicNoWind/Nonlinear Transformation ==
  data: Pc input; Vc input; OmeagC input; Rc input; P input; V input; Omega input; R input; Ve output; Oe output; Le output; Pe output
function [Ve,Oe,Le,Pe] = Nonlinear_Transformation(Pc,Vc,OmeagC,Rc,P,V,Omega,R)

Ve = V - Vc;
Oe = Omega - OmeagC;
Pe = P - Pc;
Re = R * Rc';

Pitch = atan2(-Re(3,1),sqrt(Re(1,1)^2 + Re(2,1)^2));
Yaw = atan2(Re(2,1)/cos(Pitch),Re(1,1)/cos(Pitch));
Roll = atan2(Re(3,2)/cos(Pitch),Re(3,3)/cos(Pitch));
Le = [Roll;Pitch;Yaw];

end

== matlab function QRotorSimulation/BasicNoWind/Quardrotor/MATLAB Function ==
  data: R input; dRdt output; Omega input
function dRdt = CompdRdt(R,Omega)
dRdt=R*skew(Omega);
end

== matlab function QRotorSimulation/BasicNoWind/Quardrotor/MATLAB Function1 ==
  data: R input; dPdt output; v input
function dPdt = CompdPdt(R,v)
dPdt=R*v;
end

== matlab function QRotorSimulation/BasicNoWind/Quardrotor/MATLAB Function2 ==
  data: v input; Omega input; dvdt output; Thrust input; Torque input; dOmegadt output; R input; Wx input; Wy input
function [dvdt,dOmegadt] = Dynamics(v,Omega,Thrust,Torque,R,Wx,Wy)

m = 0.25;
g = 9.8;
I = 0.1 * eye(3);
Wind = [Wx;Wy;0];
F = - Thrust * [0;0;1] + m * g * R'*[0;0;1] + Wind;


dvdt = -skew(Omega)*v + 1/m * F;
dOmegadt = -I^-1 * skew(Omega) * I * Omega + I^-1 * Torque ;

end

== matlab function QRotorSimulation/BasicNoWind/Target Generator/LambdaF ==
  data: R input; Lambda output
function Lambda = R_to_Lambda(R)

Pitch = atan2(-R(3,1),sqrt(R(1,1)^2 + R(2,1)^2));
Yaw = atan2(R(2,1)/cos(Pitch),R(1,1)/cos(Pitch));
Roll = atan2(R(3,2)/cos(Pitch),R(3,3)/cos(Pitch));
Lambda = [Roll;Pitch;Yaw];

end

== matlab function QRotorSimulation/BasicNoWind/Target Generator/MATLAB Function ==
  data: R input; dRdt output; Omega input
function dRdt = CompdRdt(R,Omega)
dRdt=R*skew(Omega);
end

== matlab function QRotorSimulation/BasicNoWind/Target Generator/MATLAB Function1 ==
  data: v input; Vc output; t input
function Vc = VcGen(v,t)
Vc = [0;0;0];

if(t>10)
    Vc = [v;0;0];
end
if(t>30)
    Vc = [0;v;0];
end

if(t>50)
    Vc = [-v;0;0];
end

if(t>70)
    Vc = [0;-v;0]; 
end

if(t>90)
    Vc = [0;0;0]; %stop
end

end

== matlab function QRotorSimulation/BasicNoWind/Target Generator/V ==
  data: R input; dPdt output; v input
function dPdt = CompdPdt(R,v)
dPdt=R*v;
end

== matlab function QRotorSimulation/Intergter/Quardrotor/MATLAB Function1 ==
  data: R input; dPdt output; v input
function dPdt = CompdPdt(R,v)
dPdt=R*v;
end

== matlab function QRotorSimulation/VObserver/Controller/Controller ==
  data: Ve input; Oe input; Le input; Pe input; Xi input; T output; n output; k input
function [T,n] = Controller(Ve,Oe,Le,Pe,Xi,k)

State = [Pe; Ve; Le; Oe;Xi];
Cntl = -k * State;
T = Cntl(1);
n = Cntl(2:4);


end

== matlab function QRotorSimulation/VObserver/Controller/Int ==
  data: Ve input; Oe input; Le input; Pe input; dXidt output
function dXidt  = Intstate(Ve,Oe,Le,Pe)
dXidt = [Pe;Le(3)];



end

== matlab function QRotorSimulation/VObserver/Nonlinear Transformation ==
  data: Pc input; Vc input; OmeagC input; Rc input; P input; V input; Omega input; R input; Ve output; Oe output; Le output; Pe output
function [Ve,Oe,Le,Pe] = Nonlinear_Transformation(Pc,Vc,OmeagC,Rc,P,V,Omega,R)

Ve = V - Vc;
Oe = Omega - OmeagC;
Pe = P - Pc;
Re = R * Rc';

Pitch = atan2(-Re(3,1),sqrt(Re(1,1)^2 + Re(2,1)^2));
Yaw = atan2(Re(2,1)/cos(Pitch),Re(1,1)/cos(Pitch));
Roll = atan2(Re(3,2)/cos(Pitch),Re(3,3)/cos(Pitch));
Le = [Roll;Pitch;Yaw];

end

== matlab function QRotorSimulation/VObserver/Quardrotor/MATLAB Function ==
  data: R input; dRdt output; Omega input
function dRdt = CompdRdt(R,Omega)
dRdt=R*skew(Omega);
end

== matlab function QRotorSimulation/VObserver/Quardrotor/MATLAB Function1 ==
  data: R input; dPdt output; v input
function dPdt = CompdPdt(R,v)
dPdt=R*v;
end

== matlab function QRotorSimulation/VObserver/Quardrotor/MATLAB Function2 ==
  data: v input; Omega input; dvdt output; Thrust input; Torque input; dOmegadt output; R input; Wx input; Wy input
function [dvdt,dOmegadt] = Dynamics(v,Omega,Thrust,Torque,R,Wx,Wy)

m = 0.25;
g = 9.8;
I = 0.1 * eye(3);
Wind = [Wx;Wy;0];
F = - Thrust * [0;0;1] + m * g * R'*[0;0;1] + Wind;


dvdt = -skew(Omega)*v + 1/m * F;
dOmegadt = -I^-1 * skew(Omega) * I * Omega + I^-1 * Torque ;

end

== matlab function QRotorSimulation/VObserver/Target Generator/LambdaF ==
  data: R input; Lambda output
function Lambda = R_to_Lambda(R)

Pitch = atan2(-R(3,1),sqrt(R(1,1)^2 + R(2,1)^2));
Yaw = atan2(R(2,1)/cos(Pitch),R(1,1)/cos(Pitch));
Roll = atan2(R(3,2)/cos(Pitch),R(3,3)/cos(Pitch));
Lambda = [Roll;Pitch;Yaw];

end

== matlab function QRotorSimulation/VObserver/Target Generator/MATLAB Function ==
  data: R input; dRdt output; Omega input
function dRdt = CompdRdt(R,Omega)
dRdt=R*skew(Omega);
end

== matlab function QRotorSimulation/Intergter/Quardrotor/MATLAB Function ==
  data: R input; dRdt output; Omega input
function dRdt = CompdRdt(R,Omega)
dRdt=R*skew(Omega);
end

== matlab function QRotorSimulation/VObserver/Target Generator/MATLAB Function1 ==
  data: v input; Vc output; t input
function Vc = VcGen(v,t)
Vc = [0;0;0];

if(t>10)
    Vc = [v;0;0];
end
if(t>30)
    Vc = [0;v;0];
end

if(t>50)
    Vc = [-v;0;0];
end

if(t>70)
    Vc = [0;-v;0]; 
end

if(t>90)
    Vc = [0;0;0]; %stop
end

end

== matlab function QRotorSimulation/VObserver/Target Generator/V ==
  data: R input; dPdt output; v input
function dPdt = CompdPdt(R,v)
dPdt=R*v;
end

== matlab function QRotorSimulation/VObserver/Observer/Controller1 ==
  data: State_est input; Oe input; Le input; Pe input; Xi input; stateEstDer output; A input; B input; C input; L input; K input; T output; n output; pest output; vest output
function [stateEstDer,T,n,pest,vest] = Observer(State_est,Oe,Le,Pe,Xi,A,B,C,L,K)


u = - K * State_est;
y = [Pe;Le;Oe;Xi];
stateEstDer = (A - L * C) * State_est + L * y + B * u;

T = u(1);
n = u(2:4);

pest = State_est(1:3);
vest = State_est(4:6);

end

== matlab function QRotorSimulation/VObserver/Observer/Int ==
  data: Ve input; Oe input; Le input; Pe input; dXidt output
function dXidt  = Intstate(Ve,Oe,Le,Pe)
dXidt = [Pe;Le(3)];



end

== matlab function QRotorSimulation/Intergter/Quardrotor/MATLAB Function2 ==
  data: v input; Omega input; dvdt output; Thrust input; Torque input; dOmegadt output; R input; Wx input; Wy input
function [dvdt,dOmegadt] = Dynamics(v,Omega,Thrust,Torque,R,Wx,Wy)

m = 0.25;
g = 9.8;
I = 0.1 * eye(3);
Wind = [Wx;Wy;0];
F = - Thrust * [0;0;1] + m * g * R'*[0;0;1] + Wind;


dvdt = -skew(Omega)*v + 1/m * F;
dOmegadt = -I^-1 * skew(Omega) * I * Omega + I^-1 * Torque ;

end

== matlab function QRotorSimulation/Intergter/Target Generator/V ==
  data: R input; dPdt output; v input
function dPdt = CompdPdt(R,v)
dPdt=R*v;
end

== matlab function QRotorSimulation/Intergter/Controller/Controller ==
  data: Ve input; Oe input; Le input; Pe input; Xi input; T output; n output; k input
function [T,n] = Controller(Ve,Oe,Le,Pe,Xi,k)

State = [Pe; Ve; Le; Oe;Xi];
Cntl = -k * State;
T = Cntl(1);
n = Cntl(2:4);


end

== matlab function QRotorSimulation/Intergter/Nonlinear Transformation ==
  data: Pc input; Vc input; OmeagC input; Rc input; P input; V input; Omega input; R input; Ve output; Oe output; Le output; Pe output
function [Ve,Oe,Le,Pe] = Nonlinear_Transformation(Pc,Vc,OmeagC,Rc,P,V,Omega,R)

Ve = V - Vc;
Oe = Omega - OmeagC;
Pe = P - Pc;
Re = R * Rc';

Pitch = atan2(-Re(3,1),sqrt(Re(1,1)^2 + Re(2,1)^2));
Yaw = atan2(Re(2,1)/cos(Pitch),Re(1,1)/cos(Pitch));
Roll = atan2(Re(3,2)/cos(Pitch),Re(3,3)/cos(Pitch));
Le = [Roll;Pitch;Yaw];

end

== matlab function QRotorSimulation/Intergter/Target Generator/LambdaF ==
  data: R input; Lambda output
function Lambda = R_to_Lambda(R)

Pitch = atan2(-R(3,1),sqrt(R(1,1)^2 + R(2,1)^2));
Yaw = atan2(R(2,1)/cos(Pitch),R(1,1)/cos(Pitch));
Roll = atan2(R(3,2)/cos(Pitch),R(3,3)/cos(Pitch));
Lambda = [Roll;Pitch;Yaw];

end
